simulink model "CTRL_UP_YTDES_test"  (R2023b)
settings: Solver=VariableStepAuto  StartTime=0.0  StopTime=10.0  RelTol=1e-3
libraries: CTRL_UP_YTDES x1
settings Model: Creator=blatak  LastModifiedBy=blatak

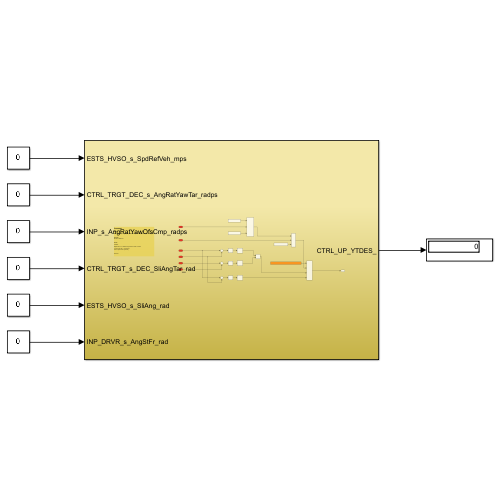
[thumbnail: Simulink's stored preview of the top-level diagram]
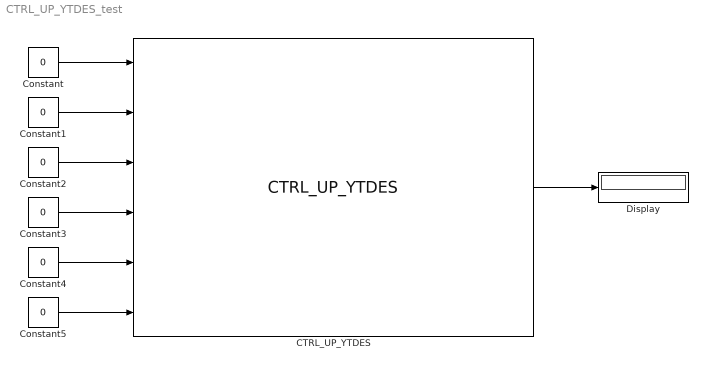
== system CTRL_UP_YTDES_test ==
  CTRL_UP_YTDES : CTRL_UP_YTDES/CTRL_UP_YTDES  SystemSampleTime=-1  VariantActivationTime=update diagram  AllowFlexibleInterface=on  Latency=0  AutoFrameSizeCalculation=off
  Constant{,1..5} (6 alike) : Constant  Value=0  OutDataTypeStr=single
  Display : Display
  wires:
  Constant/1 -> CTRL_UP_YTDES/1
  Constant1/1 -> CTRL_UP_YTDES/2
  Constant2/1 -> CTRL_UP_YTDES/3
  Constant3/1 -> CTRL_UP_YTDES/4
  Constant4/1 -> CTRL_UP_YTDES/5
  Constant5/1 -> CTRL_UP_YTDES/6
  CTRL_UP_YTDES/1 -> Display/1
